simulink model "problem4app"  (R2020a)
settings: Solver=FixedStepAuto  StartTime=0.0  StopTime=10.0  FixedStep=0.2  RelTol=1e-3
settings Model: Creator=Lenovo  LastModifiedBy=vijay
settings DataIOCC: SaveOutput=off  SaveTime=off

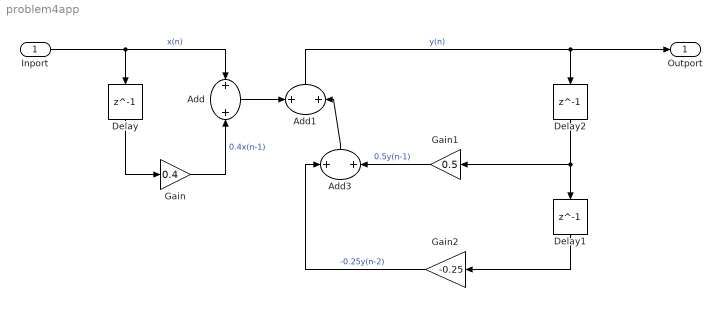
== system problem4app ==
  Inport : Inport  OutDataTypeStr=double  PortDimensions=1  SampleTime=[0.20000000000000001,0]
  Add : Sum
  Add1 : Sum
  Add3 : Sum
  Delay : Delay  DelayLength=1
  Delay1 : Delay  DelayLength=1
  Delay2 : Delay  DelayLength=1
  Gain : Gain  Gain=0.4
  Gain1 : Gain  Gain=0.5
  Gain2 : Gain  Gain=-0.25
  Outport : Outport  OutDataTypeStr=double  PortDimensions=1  SampleTime=[0.20000000000000001,0]
  wires:
  Add1/1 -> Delay2/1, Outport/1  "y(n)"
  Add/1 -> Add1/1
  Inport/1 -> Delay/1, Add/1  "x(n)"
  Delay2/1 -> Gain1/1, Delay1/1
  Delay1/1 -> Gain2/1
  Gain/1 -> Add/2  "0.4x(n-1)"
  Gain2/1 -> Add3/1  "-0.25y(n-2)"
  Gain1/1 -> Add3/2  "0.5y(n-1)"
  Add3/1 -> Add1/2
  Delay/1 -> Gain/1
